simulink model "simTwoMass"  (Simulink 9.1)
settings: Solver=ode45  StartTime=0.0  StopTime=3  RelTol=1e-3  EnableMultiTasking=on
values from neighbouring files (symbols this model uses):
  Jl = (1-q) * 2.0    (= 1.8)    [TwoMass.m]
  Jm = q * 2.0    (= 0.2)    [TwoMass.m]
  Ki = Ki*Jm*wa^2/q    [TwoMass.m]
  Kp = Kp*Jm*wa/q    [TwoMass.m]
  Ks = 100.0    (= 100)    [TwoMass.m]
settings Model: Creator=chbma  LastModifiedBy=Yu  ExtModeTrigMode=oneshot  ExtModeArmWhenConnect=off
settings DataIOCC: SignalLoggingSaveFormat=ModelDataLogs
settings OptimizationCC: BlockReduction=off  BooleanDataType=off  ExpressionDepthLimit=2147483647
settings DebuggingCC: SaveWithParameterizedLinksMsg=none  SignalResolutionControl=TryResolveAllWithWarning  MultiTaskDSMMsg=warning  MultiTaskCondExecSysMsg=none  FcnCallInpInsideContextMsg=warning  StateNameClashWarn=warning
settings HardwareCC: TargetUnknown=on
settings GRTTargetCC: GeneratePreprocessorConditionals=Disable all

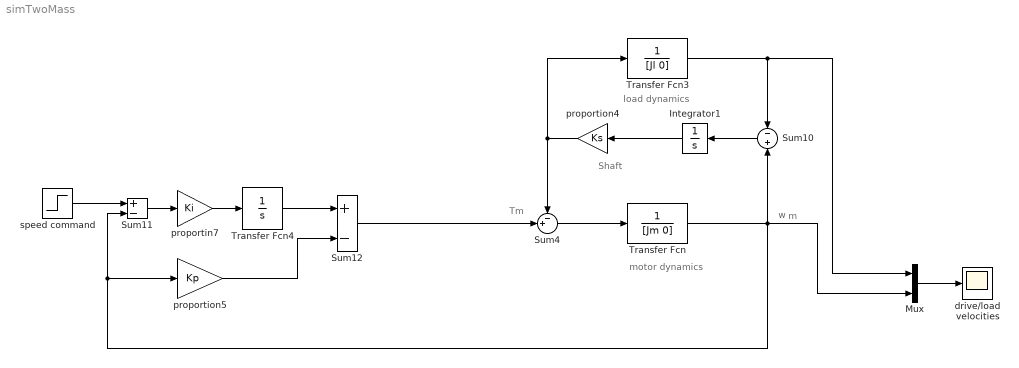
== system simTwoMass ==
  note: w
  note: Tm
  note: m
  note: motor dynamics
  note: load dynamics
  note: Shaft
  Integrator1 : Integrator
  Mux : Mux  Inputs=2
  Sum10 : Sum  Inputs=-|+  SaturateOnIntegerOverflow=on  InputSameDT=on  OutDataTypeStr=Inherit: Same as first input
  Sum11 : Sum  Inputs=+-  SaturateOnIntegerOverflow=on  InputSameDT=on  OutDataTypeStr=Inherit: Same as first input
  Sum12 : Sum  Inputs=+-  SaturateOnIntegerOverflow=on  InputSameDT=on  OutDataTypeStr=Inherit: Same as first input
  Sum4 : Sum  Inputs=-+|  SaturateOnIntegerOverflow=on  InputSameDT=on  OutDataTypeStr=Inherit: Same as first input
  Transfer Fcn : TransferFcn  Denominator=[Jm 0]
  Transfer Fcn3 : TransferFcn  Denominator=[Jl 0]
  Transfer Fcn4 : TransferFcn  Denominator=[1 0]
  drive/load velocities : Scope
  proportin7 : Gain  Gain=Ki  SaturateOnIntegerOverflow=on  OutDataTypeStr=Inherit: Same as input  ParamDataTypeStr=Inherit: Same as input
  proportion4 : Gain  Gain=Ks  SaturateOnIntegerOverflow=on  OutDataTypeStr=Inherit: Same as input  ParamDataTypeStr=Inherit: Same as input
  proportion5 : Gain  Gain=Kp  SaturateOnIntegerOverflow=on  OutDataTypeStr=Inherit: Same as input  ParamDataTypeStr=Inherit: Same as input
  speed command : Step  Time=0  After=40  SampleTime=0
  wires:
  Transfer Fcn4/1 -> Sum12/1
  proportion5/1 -> Sum12/2
  Transfer Fcn/1 -> Mux/2, Sum10/2, Sum11/2, proportion5/1
  Sum4/1 -> Transfer Fcn/1
  Transfer Fcn3/1 -> Mux/1, Sum10/1
  proportin7/1 -> Transfer Fcn4/1
  speed command/1 -> Sum11/1
  Sum11/1 -> proportin7/1
  Sum12/1 -> Sum4/2
  Integrator1/1 -> proportion4/1
  Sum10/1 -> Integrator1/1
  proportion4/1 -> Transfer Fcn3/1, Sum4/1
  Mux/1 -> drive/load velocities/1
